simulink model "Pendulums"  (R2016a)
settings: Solver=VariableStepAuto  StartTime=0.0  StopTime=10.0  RelTol=1e-3
values from neighbouring files (symbols this model uses):
  b0 = 0.15    [PendulumParameter.m]    (also in PendulumParameterT.m)
  b1 = 0.005    [PendulumParameter.m]    (also in PendulumParameter1.m; PendulumParameterT.m)
  b2 = 0.005    [PendulumParameter.m]    (also in PendulumParameter1.m; PendulumParameterT.m)
  g = 9.81    [LQRControllerPrevious.m]    (also in PendulumParameter.m; PendulumParameter1.m)
  I1 = I10+m1*(R1^2)    (= 0.00365625)    [LQRControllerPrevious.m]    (also in PendulumParameter.m = 0.624; PendulumParameter1.m = 0.624; PendulumParameterT.m)
  I2 = I20+m2*(R2^2)    (= 0.00325)    [LQRControllerPrevious.m]    (also in PendulumParameter.m = 0.624; PendulumParameter1.m = 0.624; PendulumParameterT.m)
  K = lqr(A,B,Q,R)    [LQRController.m]    (also in LQRControllerPrevious.m = lqr(sys,Q,R))
  L1 = 0.15    [LQRControllerPrevious.m]    (also in PendulumParameter.m = 2.4; PendulumParameter1.m = 2.4; PendulumParameterT.m)
  L2 = 0.2    [LQRControllerPrevious.m]    (also in PendulumParameter.m = 2.4; PendulumParameter1.m = 2.4; PendulumParameterT.m)
  m0 = 0.67    [LQRControllerPrevious.m]    (also in PendulumParameter.m = 5; PendulumParameterT.m)
  m1 = 0.15    [LQRControllerPrevious.m]    (also in PendulumParameter.m = 0.1; PendulumParameter1.m = 0.1; PendulumParameterT.m)
  m2 = 0.075    [LQRControllerPrevious.m]    (also in PendulumParameter.m = 0.1; PendulumParameter1.m = 0.1; PendulumParameterT.m)
undefined symbols (not defined in the file or in its folder): L
settings Model: Creator=VAIO  LastModifiedBy=VAIO

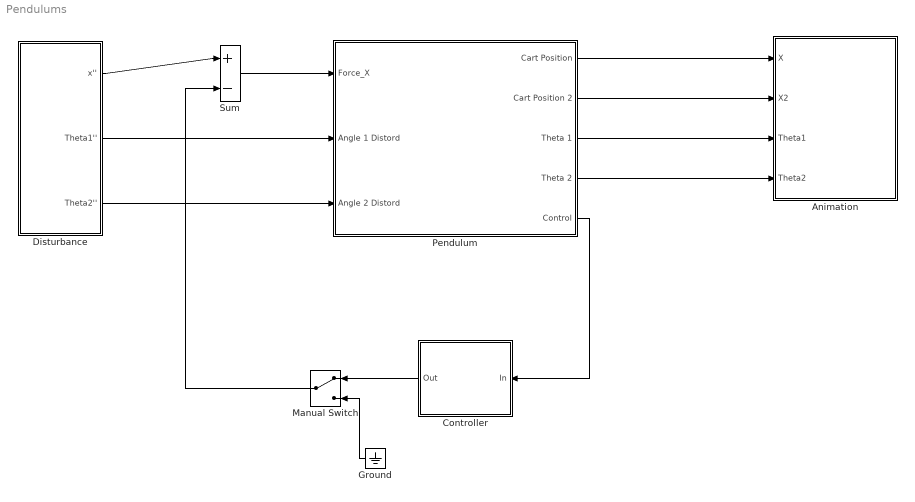
== system Pendulums ==
  Animation : Subsystem
  Controller : Subsystem
  Disturbance : Subsystem
  Ground : Ground
  Manual Switch : ManualSwitch
  Pendulum : Subsystem
  Sum : Sum  Inputs=|+-
  wires:
  Pendulum/1(Cart Position) -> Animation/1(X)
  Pendulum/2(Cart Position 2) -> Animation/2(X2)
  Pendulum/3(Theta 1) -> Animation/3(Theta1)
  Pendulum/4(Theta 2) -> Animation/4(Theta2)
  Pendulum/5(Control) -> Controller/1(In)
  Controller/1(Out) -> Manual Switch/1
  Ground/1 -> Manual Switch/2
  Sum/1 -> Pendulum/1(Force_X)
  Disturbance/1(x'') -> Sum/1
  Manual Switch/1 -> Sum/2
  Disturbance/2(Theta1'') -> Pendulum/2(Angle 1 Distord)
  Disturbance/3(Theta2'') -> Pendulum/3(Angle 2 Distord)

== system Pendulums/Animation ==
  X : Inport
  X2 : Inport  Port=2
  Theta1 : Inport  Port=3
  Theta2 : Inport  Port=4

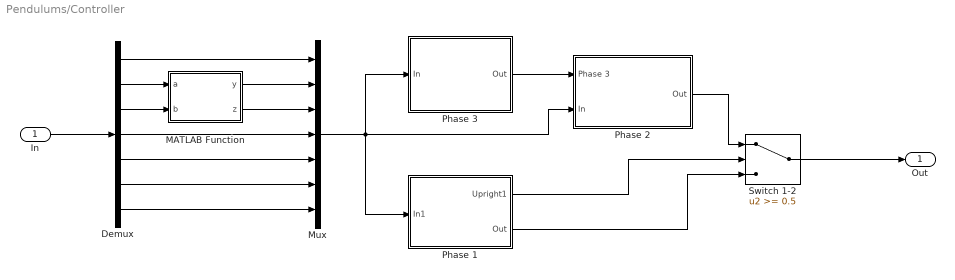
== system Pendulums/Controller ==
  In : Inport
  Demux : Demux  Outputs=7
  MATLAB Function : MATLAB Function  TreatAsAtomicUnit=on
  Mux : Mux  Inputs=7
  Phase 1 : Subsystem
  Phase 2 : Subsystem
  Phase 3 : Subsystem
  Switch 1-2 : Switch  Threshold=0.5
  Out : Outport
  wires:
  Demux/2 -> MATLAB Function/1(a)
  Demux/3 -> MATLAB Function/2(b)
  Demux/1 -> Mux/1
  MATLAB Function/1(y) -> Mux/2
  MATLAB Function/2(z) -> Mux/3
  Demux/4 -> Mux/4
  Demux/5 -> Mux/5
  Demux/6 -> Mux/6
  Demux/7 -> Mux/7
  In/1 -> Demux/1
  Mux/1 -> Phase 1/1(In1), Phase 2/2(In), Phase 3/1(In)
  Phase 3/1(Out) -> Phase 2/1(Phase 3)
  Phase 1/1(Upright1) -> Switch 1-2/2
  Phase 1/2(Out) -> Switch 1-2/3
  Phase 2/1(Out) -> Switch 1-2/1
  Switch 1-2/1 -> Out/1

== system Pendulums/Disturbance ==
  Acceleration : Constant  Value=20
  Keyboard Function : MATLAB Function  TreatAsAtomicUnit=on
  S-Function : S-Function  FunctionName=sfun_keyboard_input_v1_01  Parameters=0.01  SFunctionDeploymentMode=off  EnableBusSupport=off
  x'' : Outport
  Theta1'' : Outport  Port=2
  Theta2'' : Outport  Port=3
  wires:
  S-Function/1 -> Keyboard Function/1(d)
  Acceleration/1 -> Keyboard Function/2(a)
  Keyboard Function/3(t2) -> Theta2''/1
  Keyboard Function/2(t1) -> Theta1''/1
  Keyboard Function/1(x) -> x''/1

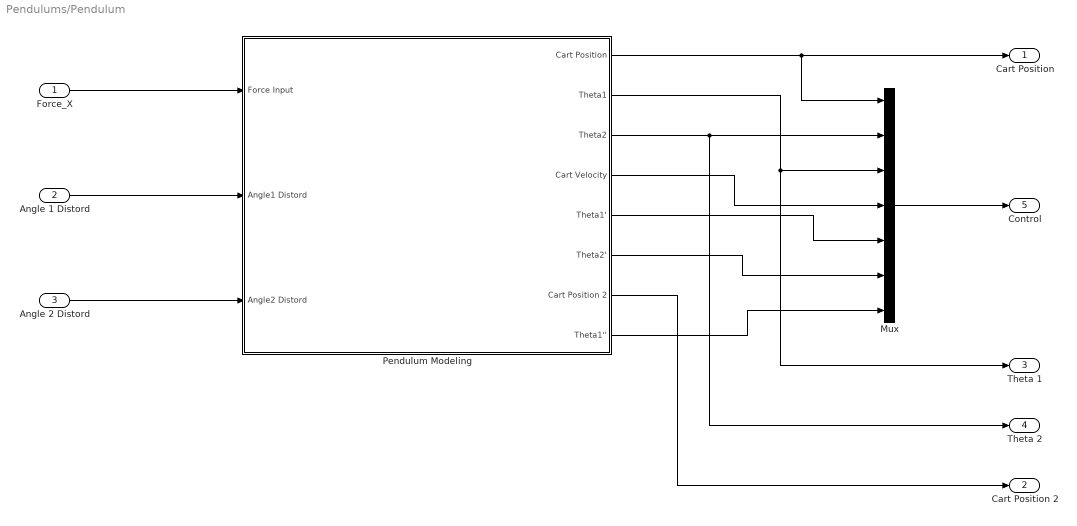
== system Pendulums/Pendulum ==
  Force_X : Inport
  Angle 1 Distord : Inport  Port=2
  Angle 2 Distord : Inport  Port=3
  Mux : Mux  Inputs=7
  Pendulum Modeling : Subsystem
  Cart Position : Outport
  Cart Position 2 : Outport  Port=2
  Theta 1 : Outport  Port=3
  Theta 2 : Outport  Port=4
  Control : Outport  Port=5
  wires:
  Force_X/1 -> Pendulum Modeling/1(Force Input)
  Angle 2 Distord/1 -> Pendulum Modeling/3(Angle2 Distord)
  Angle 1 Distord/1 -> Pendulum Modeling/2(Angle1 Distord)
  Pendulum Modeling/1(Cart Position) -> Mux/1, Cart Position/1
  Mux/1 -> Control/1
  Pendulum Modeling/2(Theta1) -> Theta 1/1, Mux/3
  Pendulum Modeling/3(Theta2) -> Theta 2/1, Mux/2
  Pendulum Modeling/4(Cart Velocity) -> Mux/4
  Pendulum Modeling/8(Theta1'') -> Mux/7
  Pendulum Modeling/7(Cart Position 2) -> Cart Position 2/1
  Pendulum Modeling/6(Theta2') -> Mux/6
  Pendulum Modeling/5(Theta1') -> Mux/5

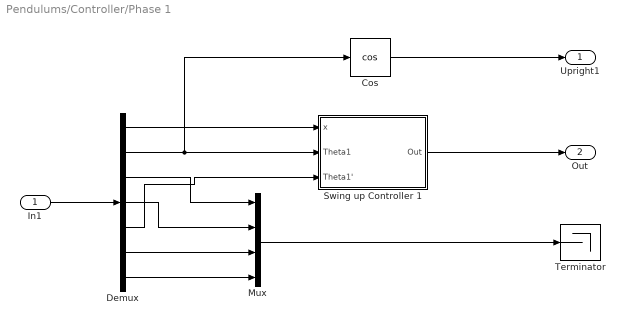
== system Pendulums/Controller/Phase 1 ==
  In1 : Inport
  Cos : Trigonometry  Operator=cos  NumberOfIterations=15
  Demux : Demux  Outputs=7
  Mux : Mux
  Swing up Controller 1 : Subsystem
  Terminator : Terminator
  Upright1 : Outport
  Out : Outport  Port=2
  wires:
  In1/1 -> Demux/1
  Demux/3 -> Mux/1
  Demux/4 -> Mux/2
  Demux/6 -> Mux/3
  Demux/7 -> Mux/4
  Cos/1 -> Upright1/1
  Mux/1 -> Terminator/1
  Demux/1 -> Swing up Controller 1/1(x)
  Swing up Controller 1/1(Out) -> Out/1
  Demux/2 -> Cos/1, Swing up Controller 1/2(Theta1)
  Demux/5 -> Swing up Controller 1/3(Theta1')

== system Pendulums/Controller/Phase 2 ==
  Phase 3 : Inport
  In : Inport  Port=2
  Gain : Gain
  MATLAB Function : MATLAB Function  TreatAsAtomicUnit=on
  Stabilizer Controller 1 : Subsystem
  Sum : Sum  Inputs=|++
  Swing up Controller 2 : Subsystem
  Out : Outport
  wires:
  MATLAB Function/1(u) -> Out/1
  Gain/1 -> Sum/1
  Sum/1 -> MATLAB Function/2(u2)
  Phase 3/1 -> MATLAB Function/1(u3)
  Stabilizer Controller 1/1(Out) -> Gain/1
  In/1 -> Swing up Controller 2/1(In), Stabilizer Controller 1/1(In)
  Swing up Controller 2/1(Out) -> Sum/2
  Swing up Controller 2/2(Theta2) -> MATLAB Function/3(t1)
  Swing up Controller 2/3(Theta2') -> MATLAB Function/4(t2)

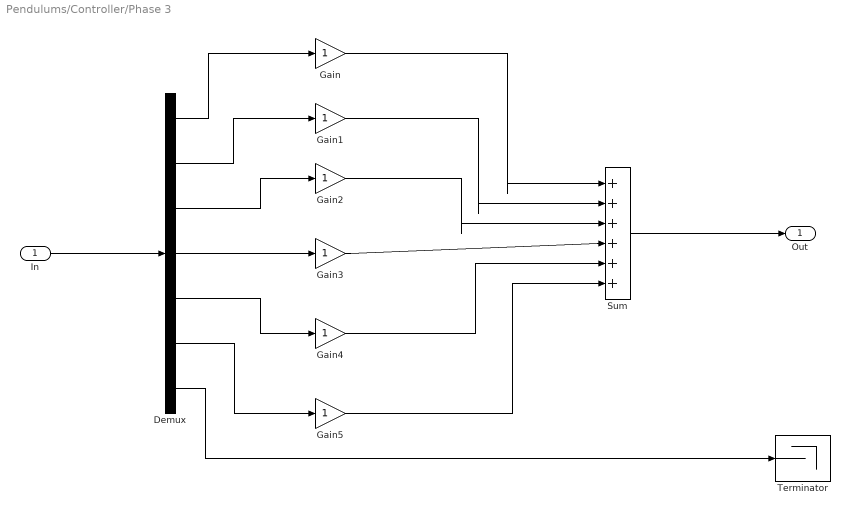
== system Pendulums/Controller/Phase 3 ==
  In : Inport
  Demux : Demux  Outputs=7
  Gain{,1..5} (6 alike) : Gain
  Sum : Sum  Inputs=|++++++
  Terminator : Terminator
  Out : Outport
  wires:
  In/1 -> Demux/1
  Demux/1 -> Gain/1
  Demux/2 -> Gain1/1
  Demux/3 -> Gain2/1
  Demux/4 -> Gain3/1
  Demux/5 -> Gain4/1
  Demux/6 -> Gain5/1
  Sum/1 -> Out/1
  Gain/1 -> Sum/1
  Gain1/1 -> Sum/2
  Gain2/1 -> Sum/3
  Gain3/1 -> Sum/4
  Gain4/1 -> Sum/5
  Gain5/1 -> Sum/6
  Demux/7 -> Terminator/1

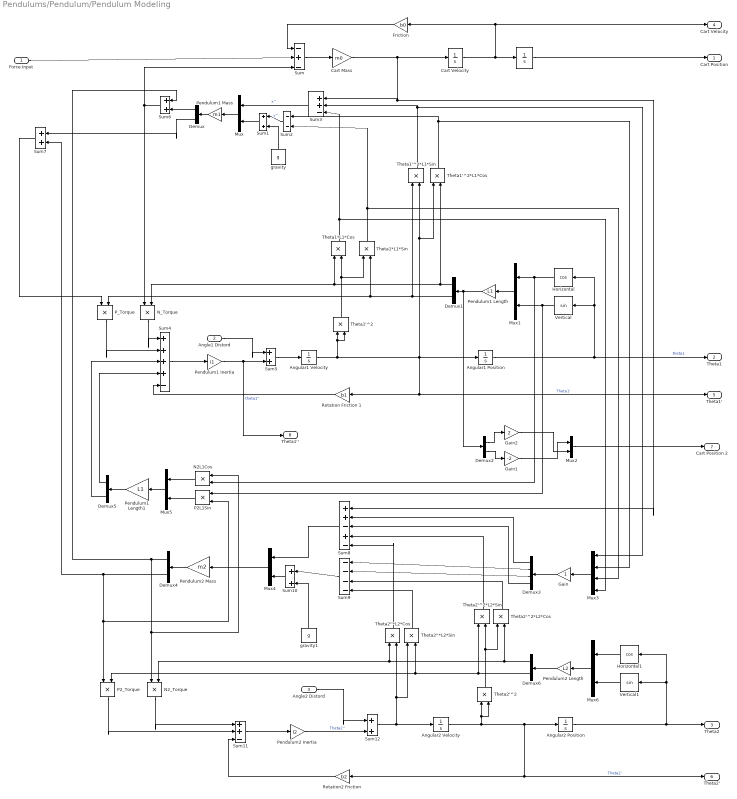
== system Pendulums/Pendulum/Pendulum Modeling ==
  Force Input : Inport
  Angle1 Distord : Inport  Port=2
  Angle2 Distord : Inport  Port=3
  " " : Integrator
  "  Vertical" : Trigonometry  NumberOfIterations=15
  "  Vertical1" : Trigonometry  NumberOfIterations=15
  Angular1 Velocity : Integrator
  Angular1 Position : Integrator
  Angular2 Position : Integrator
  Angular2 Velocity : Integrator
  Cart Velocity : Integrator
  Cart Mass : Gain  Gain=m0
  Demux{,1..2,4..6} (6 alike) : Demux  Outputs=2
  Demux3 : Demux
  Friction : Gain  Gain=b0
  Gain : Gain
  Gain1 : Gain  Gain=-2
  Gain2 : Gain  Gain=2
  "Horizontal  " : Trigonometry  Operator=cos  NumberOfIterations=15
  Horizontal1 : Trigonometry  Operator=cos  NumberOfIterations=15
  Mux{,1..2,4..6} (6 alike) : Mux  Inputs=2
  Mux3 : Mux
  N2L1Cos : Product
  N2_Torque : Product
  N_Torque : Product
  P2L1Sin : Product
  P2_Torque : Product
  P_Torque : Product
  Pendulum1 Mass : Gain  Gain=m1
  Pendulum1 Inertia : Gain  Gain=I1
  Pendulum1 Length : Gain  Gain=L1
  Pendulum1 Length1 : Gain  Gain=L1
  Pendulum2 Length : Gain  Gain=L2
  Pendulum2 Mass : Gain  Gain=m2
  Pendulum2 Inertia : Gain  Gain=I2
  Rotation Friction 1 : Gain  Gain=b1
  Rotation2 Friction : Gain  Gain=b2
  Sum : Sum  Inputs=|-+-
  Sum{1,5..7,10,12} (6 alike) : Sum  Inputs=|++
  Sum11 : Sum  Inputs=|++-
  Sum2 : Sum  Inputs=|--
  Sum3 : Sum  Inputs=|++-
  Sum4 : Sum  Inputs=|++++-
  Sum8 : Sum  Inputs=|++-+-
  Sum9 : Sum  Inputs=|----
  Theta1'^2 : Product
  Theta1'^2*L1*Cos : Product
  Theta1'^2*L1*Sin : Product
  Theta1*L1*Cos : Product
  Theta1*L1*Sin : Product
  Theta2''*L2*Cos : Product
  Theta2''*L2*Sin : Product
  Theta2'^2 : Product
  Theta2'^2*L2*Cos : Product
  Theta2'^2*L2*Sin : Product
  gravity : Constant  Value=g
  gravity1 : Constant  Value=g
  Cart Position : Outport
  Theta1 : Outport  Port=2
  Theta2 : Outport  Port=3
  Cart Velocity : Outport  Port=4
  Theta1' : Outport  Port=5
  Theta2' : Outport  Port=6
  Cart Position 2 : Outport  Port=7
  Theta1'' : Outport  Port=8
  wires:
  Force Input/1 -> Sum/2
  Sum/1 -> Cart Mass/1
  Cart Velocity/1 -> Friction/1, Cart Velocity/1, " "/1
  " "/1 -> Cart Position/1
  Friction/1 -> Sum/1
  Pendulum1 Mass/1 -> Demux/1
  Mux/1 -> Pendulum1 Mass/1
  Sum1/1 -> Mux/2
  gravity/1 -> Sum1/2
  Sum2/1 -> Sum1/1  "y''"
  Sum3/1 -> Mux/1  "x''"
  Mux1/1 -> Pendulum1 Length/1
  "  Vertical"/1 -> P2L1Sin/1, Mux1/2
  "Horizontal  "/1 -> Mux1/1, N2L1Cos/2
  Pendulum1 Length/1 -> Demux2/1, Demux1/1
  Sum4/1 -> Pendulum1 Inertia/1
  Angle1 Distord/1 -> Sum5/1
  Pendulum1 Inertia/1 -> Theta1''/1, Sum5/2  "theta1''"
  Angular1 Velocity/1 -> Theta1'^2/2, Theta1'^2/1, Angular1 Position/1, Theta1'/1, Rotation Friction 1/1, Theta1'^2*L1*Cos/1, Theta1'^2*L1*Sin/2  "Theta1'"
  Angular1 Position/1 -> "Horizontal  "/1, "  Vertical"/1, Theta1/1  "theta1"
  Rotation Friction 1/1 -> Sum4/5
  Demux2/2 -> Gain1/1
  Demux2/1 -> Gain2/1
  Gain2/1 -> Mux2/2
  Gain1/1 -> Mux2/1
  Mux2/1 -> Cart Position 2/1
  N_Torque/1 -> Sum4/1
  P_Torque/1 -> Sum4/2
  Demux1/2 -> Theta1'^2*L1*Sin/1, Theta1*L1*Sin/2, P_Torque/2
  Demux1/1 -> Theta1'^2*L1*Cos/2, Theta1*L1*Cos/1, N_Torque/2
  Demux/1 -> Sum6/2
  Sum6/1 -> Sum/3, N_Torque/1
  Demux/2 -> Sum7/1
  Sum7/1 -> P_Torque/1
  Sum5/1 -> Angular1 Velocity/1
  Mux3/1 -> Gain/1
  Cart Mass/1 -> Cart Velocity/1, Sum8/1, Sum3/1
  Theta1'^2*L1*Sin/1 -> Sum3/2, Mux3/1
  Theta1'^2*L1*Cos/1 -> Sum2/1, Mux3/2
  Theta1*L1*Sin/1 -> Sum2/2, Mux3/3
  Theta1*L1*Cos/1 -> Mux3/4, Sum3/3
  Theta1'^2/1 -> Theta1*L1*Sin/1, Theta1*L1*Cos/2
  Gain/1 -> Demux3/1
  Demux3/2 -> Sum9/1
  Demux3/3 -> Sum9/2
  Demux3/4 -> Sum8/3
  Demux3/1 -> Sum8/2
  Sum9/1 -> Sum10/1
  gravity1/1 -> Sum10/2
  Sum10/1 -> Mux4/2
  Sum8/1 -> Mux4/1
  Mux4/1 -> Pendulum2 Mass/1
  Pendulum2 Mass/1 -> Demux4/1
  Demux4/1 -> N2_Torque/1, N2L1Cos/1, Sum6/1
  Mux5/1 -> Pendulum1 Length1/1
  Pendulum1 Length1/1 -> Demux5/1
  P2L1Sin/1 -> Mux5/2
  N2L1Cos/1 -> Mux5/1
  Demux5/1 -> Sum4/4
  Demux5/2 -> Sum4/3
  Horizontal1/1 -> Mux6/1
  "  Vertical1"/1 -> Mux6/2
  Mux6/1 -> Pendulum2 Length/1
  Pendulum2 Length/1 -> Demux6/1
  Angular2 Position/1 -> "  Vertical1"/1, Horizontal1/1, Theta2/1
  Angular2 Velocity/1 -> Theta2'^2/2, Theta2'^2/1, Rotation2 Friction/1, Theta2'/1, Angular2 Position/1  "Theta2'"
  Sum12/1 -> Angular2 Velocity/1, Theta2''*L2*Sin/1, Theta2''*L2*Cos/2
  Pendulum2 Inertia/1 -> Sum12/2  "Theta2''"
  Angle2 Distord/1 -> Sum12/1
  Sum11/1 -> Pendulum2 Inertia/1
  Rotation2 Friction/1 -> Sum11/3
  N2_Torque/1 -> Sum11/1
  P2_Torque/1 -> Sum11/2
  Demux6/2 -> Theta2'^2*L2*Sin/1, Theta2''*L2*Sin/2, P2_Torque/2
  Demux6/1 -> Theta2'^2*L2*Cos/2, N2_Torque/2, Theta2''*L2*Cos/1
  Theta2'^2/1 -> Theta2'^2*L2*Cos/1, Theta2'^2*L2*Sin/2
  Theta2'^2*L2*Cos/1 -> Sum9/3
  Theta2'^2*L2*Sin/1 -> Sum8/4
  Theta2''*L2*Sin/1 -> Sum9/4
  Theta2''*L2*Cos/1 -> Sum8/5
  Demux4/2 -> P2_Torque/1, P2L1Sin/2, Sum7/2

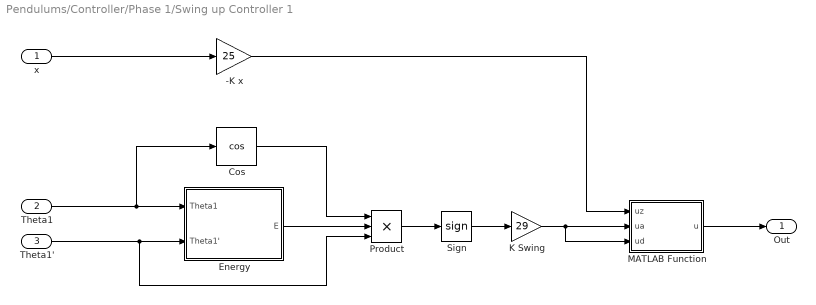
== system Pendulums/Controller/Phase 1/Swing up Controller 1 ==
  x : Inport
  Theta1 : Inport  Port=2  LockScale=on
  Theta1' : Inport  Port=3
  -K x : Gain  Gain=25
  Cos : Trigonometry  Operator=cos  NumberOfIterations=15
  Energy : Subsystem
  K Swing : Gain  Gain=29
  MATLAB Function : MATLAB Function  TreatAsAtomicUnit=on
  Product : Product  Inputs=3
  Sign : Signum
  Out : Outport
  wires:
  MATLAB Function/1(u) -> Out/1
  Sign/1 -> K Swing/1
  K Swing/1 -> MATLAB Function/3(ud), MATLAB Function/2(ua)
  Product/1 -> Sign/1
  x/1 -> -K x/1
  Theta1/1 -> Cos/1, Energy/1(Theta1)
  Theta1'/1 -> Product/3, Energy/2(Theta1')
  Energy/1(E) -> Product/2
  Cos/1 -> Product/1
  -K x/1 -> MATLAB Function/1(uz)

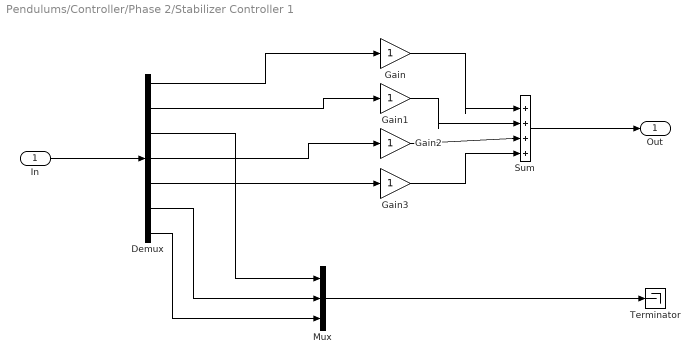
== system Pendulums/Controller/Phase 2/Stabilizer Controller 1 ==
  In : Inport
  Demux : Demux  Outputs=7
  Gain{,1..3} (4 alike) : Gain
  Mux : Mux  Inputs=3
  Sum : Sum  Inputs=|++++
  Terminator : Terminator
  Out : Outport
  wires:
  In/1 -> Demux/1
  Gain/1 -> Sum/1
  Gain1/1 -> Sum/2
  Gain2/1 -> Sum/3
  Gain3/1 -> Sum/4
  Sum/1 -> Out/1
  Demux/1 -> Gain/1
  Demux/2 -> Gain1/1
  Demux/3 -> Mux/1
  Demux/4 -> Gain2/1
  Demux/5 -> Gain3/1
  Demux/6 -> Mux/2
  Demux/7 -> Mux/3
  Mux/1 -> Terminator/1

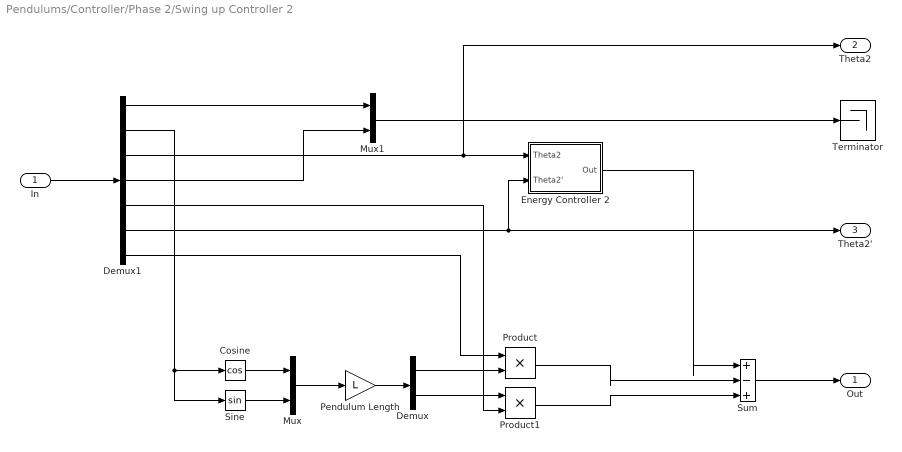
== system Pendulums/Controller/Phase 2/Swing up Controller 2 ==
  In : Inport
  Cosine : Trigonometry  Operator=cos  NumberOfIterations=15
  Demux : Demux  Outputs=2
  Demux1 : Demux  Outputs=7
  Energy Controller 2 : Subsystem
  Mux : Mux  Inputs=2
  Mux1 : Mux  Inputs=2
  Pendulum Length : Gain  Gain=L
  Product : Product
  Product1 : Product
  Sine : Trigonometry  NumberOfIterations=15
  Sum : Sum  Inputs=|+-+
  Terminator : Terminator
  Out : Outport
  Theta2 : Outport  Port=2
  Theta2' : Outport  Port=3
  wires:
  In/1 -> Demux1/1
  Demux1/1 -> Mux1/1
  Demux1/4 -> Mux1/2
  Demux1/3 -> Theta2/1, Energy Controller 2/1(Theta2)
  Product/1 -> Sum/2
  Product1/1 -> Sum/3
  Mux/1 -> Pendulum Length/1
  Pendulum Length/1 -> Demux/1
  Demux/1 -> Product/2
  Demux/2 -> Product1/1
  Demux1/7 -> Product/1
  Demux1/5 -> Product1/2
  Demux1/6 -> Energy Controller 2/2(Theta2'), Theta2'/1
  Sum/1 -> Out/1
  Energy Controller 2/1(Out) -> Sum/1
  Cosine/1 -> Mux/1
  Sine/1 -> Mux/2
  Demux1/2 -> Sine/1, Cosine/1
  Mux1/1 -> Terminator/1

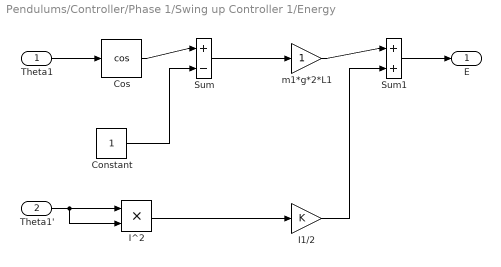
== system Pendulums/Controller/Phase 1/Swing up Controller 1/Energy ==
  Theta1 : Inport
  Theta1' : Inport  Port=2
  Constant : Constant
  Cos : Trigonometry  Operator=cos  NumberOfIterations=15
  I1/2 : Gain  Gain=K
  "I^2 " : Product
  Sum : Sum  Inputs=|+-
  Sum1 : Sum  Inputs=|++
  m1*g*2*L1 : Gain
  E : Outport
  wires:
  Theta1/1 -> Cos/1
  Cos/1 -> Sum/1
  Constant/1 -> Sum/2
  m1*g*2*L1/1 -> Sum1/1
  Sum/1 -> m1*g*2*L1/1
  Sum1/1 -> E/1
  Theta1'/1 -> "I^2 "/2, "I^2 "/1
  "I^2 "/1 -> I1/2/1
  I1/2/1 -> Sum1/2

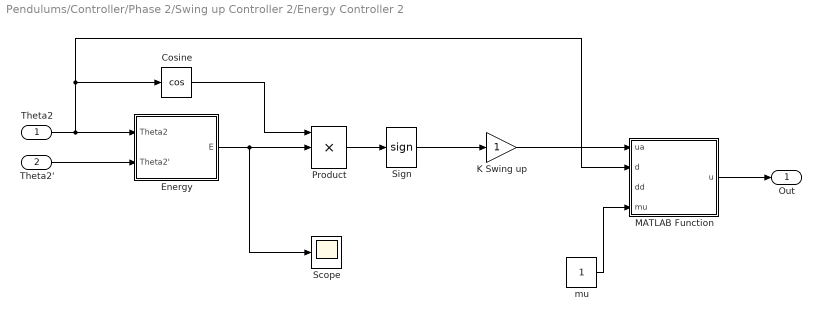
== system Pendulums/Controller/Phase 2/Swing up Controller 2/Energy Controller 2 ==
  Theta2 : Inport
  Theta2' : Inport  Port=2
  Cosine : Trigonometry  Operator=cos  NumberOfIterations=15
  Energy : Subsystem
  K Swing up : Gain
  MATLAB Function : MATLAB Function  TreatAsAtomicUnit=on
  Product : Product  Inputs=3
  Scope : Scope
  Sign : Signum
  mu : Constant
  Out : Outport
  wires:
  MATLAB Function/1(u) -> Out/1
  mu/1 -> MATLAB Function/4(mu)
  K Swing up/1 -> MATLAB Function/1(ua)
  Product/1 -> Sign/1
  Sign/1 -> K Swing up/1
  Energy/1(E) -> Scope/1, Product/2
  Theta2/1 -> Cosine/1, MATLAB Function/2(d), Energy/1(Theta2)
  Theta2'/1 -> Energy/2(Theta2')
  Cosine/1 -> Product/1

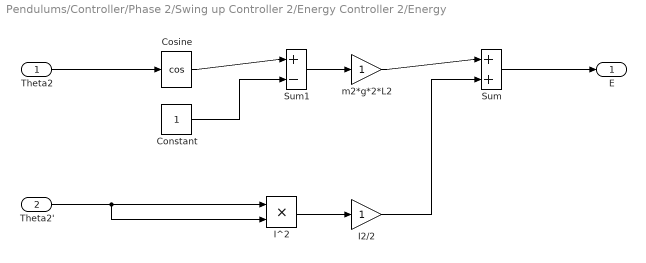
== system Pendulums/Controller/Phase 2/Swing up Controller 2/Energy Controller 2/Energy ==
  Theta2 : Inport
  Theta2' : Inport  Port=2
  Constant : Constant
  Cosine : Trigonometry  Operator=cos  NumberOfIterations=15
  I2/2 : Gain
  I^2 : Product
  Sum : Sum  Inputs=|++
  Sum1 : Sum  Inputs=|+-
  m2*g*2*L2 : Gain
  E : Outport
  wires:
  m2*g*2*L2/1 -> Sum/1
  Sum/1 -> E/1
  I^2/1 -> I2/2/1
  I2/2/1 -> Sum/2
  Sum1/1 -> m2*g*2*L2/1
  Cosine/1 -> Sum1/1
  Constant/1 -> Sum1/2
  Theta2/1 -> Cosine/1
  Theta2'/1 -> I^2/2, I^2/1

== matlab function Pendulums/Controller/Phase 1/Swing up Controller 1/MATLAB Function ==
  data: uz input; u output; ua input; ud input
function u = fcn(uz,ua,ud)

if (abs(ud)>abs(uz))||(sign(ud)==sign(uz))
    u=uz+ua;
elseif (abs(ud)<=abs(uz))&&(sign(ud)~=sign(uz))
    u=ua;
else
    u=0;
end

== matlab function Pendulums/Controller/MATLAB Function ==
  data: a input; y output; b input; z output
function [y,z] = fcn(a,b)

if a>pi
    y=a-2*pi;
elseif a<-pi
    y=a+2*pi;
else
    y=a;
end

if b>pi
    z=b-2*pi;
elseif b<-pi
    z=b+2*pi;
else
    z=b;
end

== matlab function Pendulums/Controller/Phase 2/MATLAB Function ==
  data: u3 input; u output; u2 input; t1 input; t2 input
function u = fcn(u3,u2,t1,t2)

if (cos(t1)>0.97)&&(abs(t2)<=0.5)
    u=u3;
else
    u=u2;
end

% (cos(t1)>0.955)&&(abs(t2)<=0.25)
% cos(t1)>0.97

== matlab function Pendulums/Controller/Phase 2/Swing up Controller 2/Energy Controller 2/MATLAB Function ==
  data: ua input; u output; d input; dd input; mu input
function u = fcn(ua,d,dd,mu)

if ((sin(d)*dd)<0)&&(cos(d)<cos(mu))
    u=ua;
else
    u=0;
end

== matlab function Pendulums/Disturbance/Keyboard Function ==
  data: d input; x output; a input; t1 output; t2 output
function [x,t1,t2] = fcn(d,a)

if d==28
    x=-1*a;
elseif d==29
    x=1*a;
else
    x=0;
end

if d==97
    t1=1*a;
elseif d==100
    t1=-1*a;
else
    t1=0;
end

if d==113
    t2=1*a;
elseif d==101
    t2=-1*a;
else
    t2=0;
end
